simulink model "sampleModel1930"  (R2023a)
settings: Solver=VariableStepAuto  StartTime=0.0  StopTime=10.0  RelTol=1e-3
libraries: hdlsllib x6, simulink x2
settings Model: Creator=user1  LastModifiedBy=user1

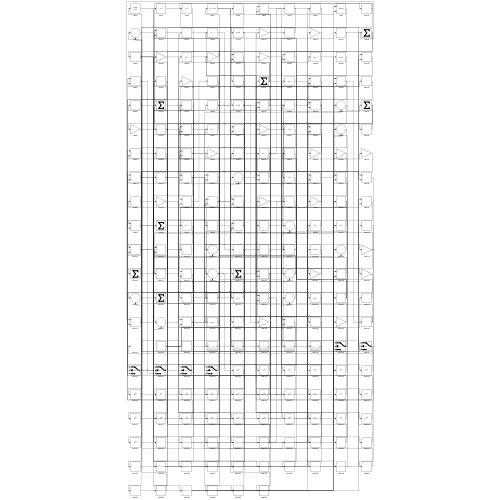
[thumbnail: Simulink's stored preview of the top-level diagram]
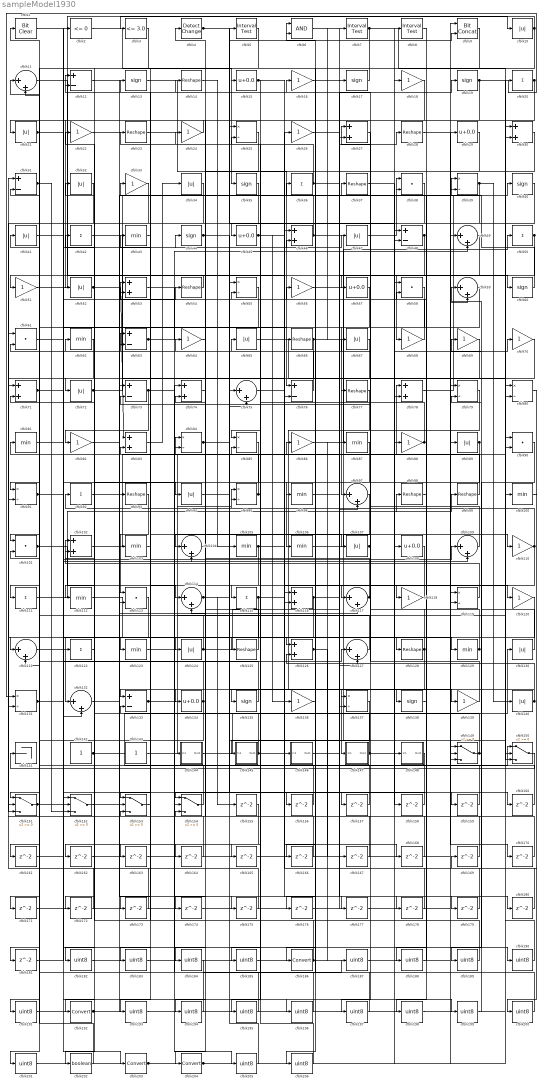
== system sampleModel1930 ==
  cfblk1 : simulink/Logic and Bit Operations/Bit Clear  iBit=0
      settings: LibrarySourceBlock=|
      | hdlsllib/Logic and Bit
      | Operations/Bit Clear
  cfblk{10,21,32,34,41,47,52,65,67,72,89,94,107,124,130,140} (16 alike) : Abs  SaturateOnIntegerOverflow=off
  cfblk{43,62,81,87,96,100,103,105..106,112,123,129} (12 alike) : MinMax
  cfblk{38,58,61,90,101,113} (6 alike) : DotProduct  OutDataTypeStr=Inherit: Inherit via internal rule
  cfblk{27,30,46,53,71,74,78,83,102,116,126} (11 alike) : Sum
  cfblk{11,49,59,75,97,104,109,114,117,121,127,132} (12 alike) : Sum  Inputs=|++
  cfblk{15,29,45,57,108,134} (6 alike) : Bias  Bias=0.0  SaturateOnIntegerOverflow=off
  cfblk{16,18,22,24,26,33,51,56,64,68..70,82,86,88,110,118,120,136,139} (20 alike) : Gain
  cfblk{20,36,42,50,92,111,115,122} (8 alike) : Sum  Inputs=+
  cfblk{25,39,55,79..80,84..85,91,95,119,131,137} (12 alike) : Product  Inputs=*/  RndMeth=Zero  SaturateOnIntegerOverflow=on
  cfblk{12,31,48,63,73,76,133} (7 alike) : Sum  Inputs=+-
  cfblk{14,23,28,37,54,66,77,93,98..99,125,128} (12 alike) : Reshape
  cfblk{13,17,19,35,40,44,60,135,138} (9 alike) : Signum
  cfblk141 : Terminator
  cfblk142 : Constant  SampleTime=-1
  cfblk143 : Constant  SampleTime=-1
  cfblk144 : Subsystem
      settings: LibrarySourceBlock=|
      | hdlsllib/Ports &
      | Subsystems/Subsystem
  cfblk145 : Subsystem
      settings: LibrarySourceBlock=|
      | hdlsllib/Ports &
      | Subsystems/Subsystem
  cfblk146 : Subsystem
      settings: LibrarySourceBlock=|
      | hdlsllib/Ports &
      | Subsystems/Subsystem
  cfblk147 : Subsystem
      settings: LibrarySourceBlock=|
      | hdlsllib/Ports &
      | Subsystems/Subsystem
  cfblk148 : Subsystem
      settings: LibrarySourceBlock=|
      | hdlsllib/Ports &
      | Subsystems/Subsystem
  cfblk{149..154} (6 alike) : Switch  SaturateOnIntegerOverflow=off  InputSameDT=off
  cfblk{155..181} (27 alike) : Delay  SampleTime=1
  cfblk{182..185,187..191,193..201,205..206} (20 alike) : DataTypeConversion  OutDataTypeStr=uint8  SaturateOnIntegerOverflow=off  RndMeth=Floor
  cfblk{186,192,203..204} (4 alike) : DataTypeConversion  SaturateOnIntegerOverflow=off  RndMeth=Floor
  cfblk2 : hdlsllib/Logic and Bit Operations/Compare To Zero  relop=<=  OutDataTypeStr=boolean
  cfblk202 : DataTypeConversion  OutDataTypeStr=boolean  SaturateOnIntegerOverflow=off  RndMeth=Floor
  cfblk3 : hdlsllib/Logic and Bit Operations/Compare To Constant  relop=<=  const=3.0  OutDataTypeStr=boolean
  cfblk4 : simulink/Logic and Bit Operations/Detect Change  vinit=0  OutDataTypeStr=boolean
      settings: LibrarySourceBlock=|
      | hdlsllib/Logic and Bit
      | Operations/Detect
      | Change
  cfblk5 : hdlsllib/Logic and Bit Operations/Interval Test  IntervalClosedRight=on  uplimit=0.5  IntervalClosedLeft=on  lowlimit=-0.5  OutDataTypeStr=boolean
  cfblk6 : Logic  AllPortsSameDT=off  OutDataTypeStr=boolean
  cfblk7 : hdlsllib/Logic and Bit Operations/Interval Test  IntervalClosedRight=on  uplimit=0.5  IntervalClosedLeft=on  lowlimit=-0.5  OutDataTypeStr=boolean
  cfblk8 : hdlsllib/Logic and Bit Operations/Interval Test  IntervalClosedRight=on  uplimit=0.5  IntervalClosedLeft=on  lowlimit=-0.5  OutDataTypeStr=boolean
  cfblk9 : hdlsllib/Logic and Bit Operations/Bit Concat  numInputs=2
  wires:
  cfblk113/1 -> cfblk121/1
  cfblk45/1 -> cfblk136/1, cfblk177/1
  cfblk14/1 -> cfblk105/1
  cfblk66/1 -> cfblk7/1, cfblk80/2, cfblk171/1
  cfblk18/1 -> cfblk192/1
  cfblk78/1 -> cfblk40/1
  cfblk83/1 -> cfblk34/1
  cfblk77/1 -> cfblk147/1(In1)
  cfblk2/1 -> cfblk35/1
  cfblk142/1 -> cfblk150/1, cfblk8/1, cfblk26/1, cfblk127/2
  cfblk23/1 -> cfblk76/1
  cfblk150/1 -> cfblk141/1
  cfblk51/1 -> cfblk10/1
  cfblk89/1 -> cfblk106/1, cfblk85/2
  cfblk120/1 -> cfblk132/1
  cfblk125/1 -> cfblk81/1
  cfblk60/1 -> cfblk33/1
  cfblk106/1 -> cfblk110/1
  cfblk15/1 -> cfblk45/1, cfblk178/1
  cfblk62/1 -> cfblk72/1
  cfblk109/1 -> cfblk65/1
  cfblk6/1 -> cfblk17/1
  cfblk17/1 -> cfblk15/1
  cfblk116/1 -> cfblk28/1, cfblk201/1
  cfblk46/1 -> cfblk150/2, cfblk36/1
  cfblk68/1 -> cfblk23/1
  cfblk10/1 -> cfblk96/1, cfblk3/1
  cfblk40/1 -> cfblk85/1
  cfblk50/1 -> cfblk135/1, cfblk113/2
  cfblk86/1 -> cfblk50/1
  cfblk13/1 -> cfblk116/1
  cfblk29/1 -> cfblk115/1
  cfblk128/1 -> cfblk12/1, cfblk173/1, cfblk174/1
  cfblk67/1 -> cfblk151/1
  cfblk9/1 -> cfblk123/1
  cfblk95/1 -> cfblk4/1, cfblk125/1
  cfblk73/1 -> cfblk126/1, cfblk112/1, cfblk205/1
  cfblk19/1 -> cfblk131/1, cfblk137/2
  cfblk52/1 -> cfblk83/1, cfblk82/1
  cfblk117/1 -> cfblk14/1, cfblk12/2
  cfblk134/1 -> cfblk102/2, cfblk191/1
  cfblk130/1 -> cfblk59/1
  cfblk88/1 -> cfblk64/1, cfblk53/2
  cfblk44/1 -> cfblk37/1, cfblk159/1
  cfblk92/1 -> cfblk84/1
  cfblk129/1 -> cfblk16/1, cfblk73/2, cfblk102/1
  cfblk118/1 -> cfblk117/1
  cfblk131/1 -> cfblk109/1, cfblk11/2
  cfblk139/1 -> cfblk92/1
  cfblk133/1 -> cfblk78/1, cfblk104/2
  cfblk115/1 -> cfblk120/1, cfblk151/3
  cfblk48/1 -> cfblk68/1, cfblk172/1
  cfblk70/1 -> cfblk97/1
  cfblk75/1 -> cfblk39/1
  cfblk59/1 -> cfblk77/1
  cfblk105/1 -> cfblk133/1, cfblk128/1
  cfblk102/1 -> cfblk30/1
  cfblk132/1 -> cfblk39/2
  cfblk110/1 -> cfblk95/1, cfblk118/1
  cfblk63/1 -> cfblk107/1, cfblk49/2
  cfblk34/1 -> cfblk153/1
  cfblk91/1 -> cfblk109/2, cfblk54/1
  cfblk93/1 -> cfblk113/1
  cfblk111/1 -> cfblk99/1
  cfblk58/1 -> cfblk186/1
  cfblk54/1 -> cfblk51/1
  cfblk143/1 -> cfblk95/2
  cfblk112/1 -> cfblk146/1(In1)
  cfblk82/1 -> cfblk117/2
  cfblk124/1 -> cfblk19/1, cfblk32/1
  cfblk21/1 -> cfblk132/2, cfblk196/1, cfblk199/1
  cfblk20/1 -> cfblk52/1, cfblk124/1
  cfblk149/1 -> cfblk71/2, cfblk69/1
  cfblk119/1 -> cfblk27/1
  cfblk98/1 -> cfblk38/1
  cfblk154/1 -> cfblk41/1
  cfblk101/1 -> cfblk114/1, cfblk46/2
  cfblk57/1 -> cfblk101/1
  cfblk25/1 -> cfblk204/1
  cfblk53/1 -> cfblk144/1(In1)
  cfblk144/1(Out1) -> cfblk130/1
  cfblk99/1 -> cfblk86/1
  cfblk145/1(Out1) -> cfblk43/1, cfblk168/1
  cfblk127/1 -> cfblk31/2
  cfblk47/1 -> cfblk38/2
  cfblk24/1 -> cfblk21/1
  cfblk76/1 -> cfblk61/2
  cfblk72/1 -> cfblk20/1, cfblk179/1
  cfblk39/1 -> cfblk140/1, cfblk195/1
  cfblk65/1 -> cfblk150/3
  cfblk135/1 -> cfblk11/1
  cfblk146/1(Out1) -> cfblk98/1
  cfblk16/1 -> cfblk138/1
  cfblk71/1 -> cfblk154/2, cfblk129/1
  cfblk11/1 -> cfblk116/2
  cfblk84/1 -> cfblk75/1, cfblk47/1
  cfblk126/1 -> cfblk166/1, cfblk167/1
  cfblk56/1 -> cfblk88/1
  cfblk81/1 -> cfblk122/1
  cfblk152/1 -> cfblk103/1
  cfblk122/1 -> cfblk42/1
  cfblk140/1 -> cfblk134/1, cfblk126/2
  cfblk104/1 -> cfblk74/2
  cfblk36/1 -> cfblk24/1, cfblk13/1, cfblk180/1
  cfblk32/1 -> cfblk131/2
  cfblk147/1(Out1) -> cfblk70/1, cfblk6/1
  cfblk107/1 -> cfblk67/1, cfblk157/1
  cfblk64/1 -> cfblk104/1
  cfblk94/1 -> cfblk139/1
  cfblk41/1 -> cfblk94/1
  cfblk38/1 -> cfblk145/1(In1)
  cfblk31/1 -> cfblk91/1, cfblk152/3
  cfblk26/1 -> cfblk60/1
  cfblk114/1 -> cfblk149/3, cfblk155/1
  cfblk22/1 -> cfblk73/1
  cfblk33/1 -> cfblk151/2
  cfblk151/1 -> cfblk44/1, cfblk127/1
  cfblk4/1 -> cfblk9/2, cfblk48/2
  cfblk123/1 -> cfblk30/2
  cfblk7/1 -> cfblk80/1, cfblk111/1
  cfblk69/1 -> cfblk91/2
  cfblk61/1 -> cfblk66/1
  cfblk1/1 -> cfblk203/1
  cfblk42/1 -> cfblk76/2
  cfblk27/1 -> cfblk57/1
  cfblk30/1 -> cfblk137/1
  cfblk103/1 -> cfblk53/1
  cfblk153/1 -> cfblk63/1
  cfblk121/1 -> cfblk156/1
  cfblk156/1 -> cfblk84/2
  cfblk157/1 -> cfblk101/2
  cfblk37/1 -> cfblk158/1
  cfblk158/1 -> cfblk154/1
  cfblk159/1 -> cfblk63/2
  cfblk96/1 -> cfblk160/1
  cfblk160/1 -> cfblk149/1
  cfblk3/1 -> cfblk161/1
  cfblk87/1 -> cfblk162/1
  cfblk162/1 -> cfblk59/2
  cfblk85/1 -> cfblk163/1
  cfblk163/1 -> cfblk83/2
  cfblk74/1 -> cfblk164/1
  cfblk164/1 -> cfblk153/3
  cfblk137/1 -> cfblk165/1
  cfblk165/1 -> cfblk97/2
  cfblk166/1 -> cfblk152/1
  cfblk167/1 -> cfblk154/3
  cfblk168/1 -> cfblk114/2
  cfblk80/1 -> cfblk169/1
  cfblk169/1 -> cfblk61/1
  cfblk28/1 -> cfblk170/1
  cfblk170/1 -> cfblk153/2
  cfblk171/1 -> cfblk48/1
  cfblk172/1 -> cfblk152/2
  cfblk173/1 -> cfblk31/1
  cfblk174/1 -> cfblk75/2
  cfblk12/1 -> cfblk175/1
  cfblk175/1 -> cfblk71/1
  cfblk136/1 -> cfblk176/1
  cfblk176/1 -> cfblk27/2
  cfblk177/1 -> cfblk119/2
  cfblk178/1 -> cfblk6/2
  cfblk179/1 -> cfblk149/2
  cfblk180/1 -> cfblk46/1
  cfblk35/1 -> cfblk181/1
  cfblk181/1 -> cfblk2/1
  cfblk5/1 -> cfblk182/1
  cfblk182/1 -> cfblk89/1
  cfblk43/1 -> cfblk183/1
  cfblk183/1 -> cfblk5/1
  cfblk148/1(Out1) -> cfblk184/1
  cfblk108/1 -> cfblk185/1
  cfblk185/1 -> cfblk148/1(In1)
  cfblk186/1 -> cfblk22/1, cfblk133/2, cfblk87/1
  cfblk184/1 -> cfblk187/1
  cfblk187/1 -> cfblk58/1
  cfblk8/1 -> cfblk188/1
  cfblk188/1 -> cfblk58/2
  cfblk90/1 -> cfblk189/1
  cfblk189/1 -> cfblk62/1
  cfblk161/1 -> cfblk190/1
  cfblk190/1 -> cfblk90/1
  cfblk191/1 -> cfblk90/2
  cfblk192/1 -> cfblk93/1, cfblk108/1
  cfblk97/1 -> cfblk193/1
  cfblk193/1 -> cfblk18/1
  cfblk55/1 -> cfblk194/1
  cfblk194/1 -> cfblk121/2
  cfblk195/1 -> cfblk55/1
  cfblk196/1 -> cfblk55/2
  cfblk79/1 -> cfblk197/1
  cfblk197/1 -> cfblk56/1
  cfblk138/1 -> cfblk198/1
  cfblk198/1 -> cfblk79/1
  cfblk199/1 -> cfblk79/2
  cfblk100/1 -> cfblk200/1
  cfblk200/1 -> cfblk74/1
  cfblk201/1 -> cfblk100/1
  cfblk155/1 -> cfblk202/1
  cfblk202/1 -> cfblk1/1
  cfblk203/1 -> cfblk29/1, cfblk49/1, cfblk119/1
  cfblk204/1 -> cfblk78/2, cfblk9/1
  cfblk205/1 -> cfblk25/1
  cfblk49/1 -> cfblk206/1
  cfblk206/1 -> cfblk25/2

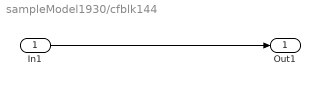
== system sampleModel1930/cfblk144 ==
  In1 : Inport
  Out1 : Outport
  wires:
  In1/1 -> Out1/1

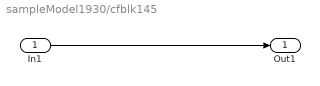
== system sampleModel1930/cfblk145 ==
  In1 : Inport
  Out1 : Outport
  wires:
  In1/1 -> Out1/1

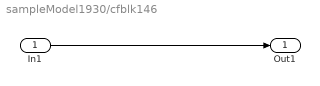
== system sampleModel1930/cfblk146 ==
  In1 : Inport
  Out1 : Outport
  wires:
  In1/1 -> Out1/1

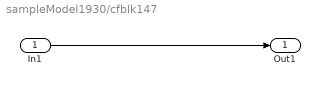
== system sampleModel1930/cfblk147 ==
  In1 : Inport
  Out1 : Outport
  wires:
  In1/1 -> Out1/1

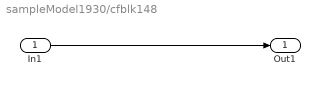
== system sampleModel1930/cfblk148 ==
  In1 : Inport
  Out1 : Outport
  wires:
  In1/1 -> Out1/1
